simulink model "MIL4L3_SW6_V1_20220211"  (R2018b)
settings: Solver=FixedStepAuto  StartTime=0.0  StopTime=inf  FixedStep=0.001  RelTol=1e-3
PreLoadFcn:
  | A0_MILtest;
undefined symbols (not defined in the file or in its folder): Clb_ICADirect_LaneDisp_StateFive, Clb_ICADirect_LaneDisp_StateFour, Clb_ICADirect_LaneDisp_StateOne, Clb_ICADirect_LaneDisp_StateThree, Clb_ICADirect_LaneDisp_StateTwo, Clb_ICADirect_LaneDisp_StateZero, Clb_ICADirect_LaneDispSW, Clb_ICADirect_TrnLghtsCom_Switch, Clb_ICADirect_TrnLghtsCom_Value, Clb_ICADirect_TrnLghtsCrtl_Inhb, IMAP_Clb_ACU_Driver_Belt, IMAP_Clb_ACU_Driver_Belt_Over, IMAP_Clb_ACU_Passenger_Belt, IMAP_Clb_ACU_Passenger_Belt_Over, IMAP_Clb_ACU_RearLeft_Belt, IMAP_Clb_ACU_RearLeft_Belt_Over, IMAP_Clb_ACU_RearMiddle_Belt, IMAP_Clb_ACU_RearMiddle_Belt_Over, IMAP_Clb_ACU_RearRight_Belt, IMAP_Clb_ACU_RearRight_Belt_Over, IMAP_Clb_AEB_Switch, IMAP_Clb_AEB_Switch_Over, IMAP_Clb_ALC_TLC_Mode, IMAP_Clb_ALC_TLC_Mode_Over, IMAP_Clb_BCM_Battery_Voltage, IMAP_Clb_BCM_Battery_Voltage_Over, IMAP_Clb_BCM_BrakeLamp_State, IMAP_Clb_BCM_BrakeLamp_State_Over, IMAP_Clb_BCM_CHMSL_Status, IMAP_Clb_BCM_CHMSL_Status_Over, IMAP_Clb_BCM_Door_Lock_State, IMAP_Clb_BCM_Door_Lock_State_Over, IMAP_Clb_BCM_FrontWiper_State, IMAP_Clb_BCM_FrontWiper_State_Over, IMAP_Clb_BCM_FrontWiper_Switch, IMAP_Clb_BCM_FrontWiper_Switch_Over, IMAP_Clb_BCM_HazardLamp, IMAP_Clb_BCM_HazardLamp_Over, IMAP_Clb_BCM_HazardLamp_Switch, IMAP_Clb_BCM_HazardLamp_Switch_Over, IMAP_Clb_BCM_HighBeam_State, IMAP_Clb_BCM_HighBeam_State_Over, IMAP_Clb_BCM_Ignition_State, IMAP_Clb_BCM_Ignition_State_Over, IMAP_Clb_BCM_IHBC_Enabled, IMAP_Clb_BCM_IHBC_Enabled_Over, IMAP_Clb_BCM_Left_Light, IMAP_Clb_BCM_Left_Light_Over, IMAP_Clb_BCM_LeftTurn_Switch, IMAP_Clb_BCM_LeftTurn_Switch_Over, IMAP_Clb_BCM_LF_Door_State, IMAP_Clb_BCM_LF_Door_State_Over, IMAP_Clb_BCM_LowBeam_State, IMAP_Clb_BCM_LowBeam_State_Over, IMAP_Clb_BCM_LR_Door_State, IMAP_Clb_BCM_LR_Door_State_Over, IMAP_Clb_BCM_RF_Door_State, IMAP_Clb_BCM_RF_Door_State_Over, IMAP_Clb_BCM_Right_Light, IMAP_Clb_BCM_Right_Light_Over ... (+547)
libraries: CarMaker4SL x2153, simulink x292, dspstat3 x3, canmsglib x2, simulink_extras x1
(part 18 of 52)

== system MIL4L3_SW6_V1_20220211/CarMaker/VehicleControl/SDFADataLog/Subsystem97 ==
  BusCreator : BusCreator  Inputs=10
  Data Type Conversion{1..3,92} (4 alike) : DataTypeConversion  OutDataTypeStr=single
  Ground{,1..5} (6 alike) : Ground
  Read CM Dict1 : CarMaker4SL/Read CM Dict  xname=User.IO.Out.ReferencePoint_S0_002  xsync=off
  Read CM Dict2 : CarMaker4SL/Read CM Dict  xname=User.IO.Out.ReferencePoint_S0_003  xsync=off
  Read CM Dict3 : CarMaker4SL/Read CM Dict  xname=User.IO.Out.ReferencePoint_S0_004  xsync=off
  Read CM Dict5 : CarMaker4SL/Read CM Dict  xname=User.IO.Out.ReferencePoint_S0_001  xsync=off
  LBtar_ReferencePoint : Outport
  wires:
  Data Type Conversion3/1 -> BusCreator/4
  Data Type Conversion2/1 -> BusCreator/3
  Data Type Conversion92/1 -> BusCreator/1
  Data Type Conversion1/1 -> BusCreator/2
  Ground5/1 -> BusCreator/10
  Ground4/1 -> BusCreator/9
  Ground3/1 -> BusCreator/8
  Ground2/1 -> BusCreator/7
  Ground1/1 -> BusCreator/6
  Ground/1 -> BusCreator/5
  Read CM Dict5/1 -> Data Type Conversion92/1
  Read CM Dict1/1 -> Data Type Conversion1/1
  Read CM Dict2/1 -> Data Type Conversion2/1
  Read CM Dict3/1 -> Data Type Conversion3/1
  BusCreator/1 -> LBtar_ReferencePoint/1

== system MIL4L3_SW6_V1_20220211/CarMaker/VehicleControl/SDFADataLog/Subsystem98 ==
  BusCreator : BusCreator  Inputs=10
  Data Type Conversion{1..3,92} (4 alike) : DataTypeConversion  OutDataTypeStr=single
  Ground{,1..5} (6 alike) : Ground
  Read CM Dict1 : CarMaker4SL/Read CM Dict  xname=User.IO.Out.MovingState_S0_002  xsync=off
  Read CM Dict2 : CarMaker4SL/Read CM Dict  xname=User.IO.Out.MovingState_S0_003  xsync=off
  Read CM Dict3 : CarMaker4SL/Read CM Dict  xname=User.IO.Out.MovingState_S0_004  xsync=off
  Read CM Dict5 : CarMaker4SL/Read CM Dict  xname=User.IO.Out.MovingState_S0_001  xsync=off
  LBtar_MovingState : Outport
  wires:
  Data Type Conversion92/1 -> BusCreator/1
  Data Type Conversion2/1 -> BusCreator/3
  Data Type Conversion3/1 -> BusCreator/4
  Data Type Conversion1/1 -> BusCreator/2
  BusCreator/1 -> LBtar_MovingState/1
  Read CM Dict3/1 -> Data Type Conversion3/1
  Read CM Dict2/1 -> Data Type Conversion2/1
  Read CM Dict1/1 -> Data Type Conversion1/1
  Read CM Dict5/1 -> Data Type Conversion92/1
  Ground/1 -> BusCreator/5
  Ground1/1 -> BusCreator/6
  Ground2/1 -> BusCreator/7
  Ground3/1 -> BusCreator/8
  Ground4/1 -> BusCreator/9
  Ground5/1 -> BusCreator/10

== system MIL4L3_SW6_V1_20220211/CarMaker/VehicleControl/SwitchForRealECU_ACC_Brake/PI Control ==
  Add : Sum
  Constant : Constant  Value=0
  Constant1 : Constant  Value=0
  Constant2 : Constant  Value=0
  Define CM Dict5 : CarMaker4SL/Define CM Dict  xname=User.IO.In.P_gain  xmono=off  xtype=Double4  xdvaplace=IO_In  xnstates=0  xfirststate=0  xinitial=-0.06
  Define CM Dict6 : CarMaker4SL/Define CM Dict  xname=User.IO.In.I_gain  xmono=off  xtype=Double4  xdvaplace=IO_In  xnstates=0  xfirststate=0  xinitial=-0.03
  Delta ax : Sum  Inputs=+-
  Memory : Memory
  Product : Product
  Product1 : Product
  Read CM Dict1 : CarMaker4SL/Read CM Dict  xname=User.IO.In.P_gain  xsync=off
  Read CM Dict2 : CarMaker4SL/Read CM Dict  xname=User.IO.In.I_gain  xsync=off
  Read CM Dict7 : CarMaker4SL/Read CM Dict  xname=Car.ax  xsync=off
  Saturation : Saturate  UpperLimit=1  LowerLimit=0
  Saturation1 : Saturate  UpperLimit=1  LowerLimit=0
  Sum : Sum  Inputs=|++
  Switch : Switch  Criteria=u2 > Threshold
  Switch1 : Switch  Criteria=u2 > Threshold
  Switch2 : Switch  Criteria=u2 > Threshold
  Out1 : Outport
  wires:
  [ADAS_DecelerationSet] -> Switch/1
  Switch/1 -> Delta ax/1
  Delta ax/1 -> Product1/1, Product/2
  Add/1 -> Saturation1/1
  Product/1 -> Add/1
  Product1/1 -> Sum/1
  Sum/1 -> Memory/1, Switch2/1
  Memory/1 -> Saturation/1
  Saturation/1 -> Sum/2
  Read CM Dict1/1 -> Product/1
  Read CM Dict2/1 -> Product1/2
  [MDD_Decelerationcontrol_request] -> Switch1/2, Switch2/2, Switch/2
  Read CM Dict7/1 -> Switch1/1
  Constant/1 -> Switch1/3
  Switch1/1 -> Delta ax/2
  Switch2/1 -> Add/2
  Constant1/1 -> Switch2/3
  Saturation1/1 -> Out1/1
  Constant2/1 -> Switch/3

== system MIL4L3_SW6_V1_20220211/CarMaker/VehicleControl/SwitchForRealECU_ACC_Gas/PI Control ==
  In1 : Inport
  Add : Sum
  Compare To Constant1 : simulink/Logic and Bit Operations/Compare To Constant  relop===  const=1  OutDataTypeStr=boolean
  Constant : Constant  Value=0
  Constant1 : Constant  Value=0
  Define CM Dict5 : CarMaker4SL/Define CM Dict  xname=User.IO.In.EngTrqManualC  xmono=off  xtype=Double4  xdvaplace=IO_In  xnstates=0  xfirststate=0  xinitial=1
  Delta Tq : Sum  Inputs=+-
  Gain : Gain  Gain=-1/500
  Gain1 : Gain  Gain=-1/500
  Gain2 : Gain  Gain=0.95
  Gain3 : Gain  Gain=0.98
  Gain4 : Gain
  Memory : Memory
  Product : Product
  Product1 : Product
  Product2 : Product  Inputs=3
  Read CM Dict1 : CarMaker4SL/Read CM Dict  xname=User.IO.In.P_gain  xsync=off
  Read CM Dict11 : CarMaker4SL/Read CM Dict  xname=PT.Engine.Trq  xsync=off
  Read CM Dict2 : CarMaker4SL/Read CM Dict  xname=User.IO.In.I_gain  xsync=off
  Read CM Dict3 : CarMaker4SL/Read CM Dict  xname=User.IO.In.ADAS_PowerWheelTorqueActiveReq  xsync=off
  Read CM Dict5 : CarMaker4SL/Read CM Dict  xname=User.IO.In.EngTrqManualC  xsync=off
  Saturation : Saturate  UpperLimit=1  LowerLimit=0
  Saturation1 : Saturate  UpperLimit=1  LowerLimit=0
  Subsystem1 : Subsystem
  Sum : Sum  Inputs=|++
  Switch1 : Switch  Criteria=u2 > Threshold  Threshold=0.5
  Switch2 : Switch  Criteria=u2 > Threshold  Threshold=0.5
  Out1 : Outport
  wires:
  In1/1 -> Delta Tq/1
  Delta Tq/1 -> Product1/1, Product/2
  Product/1 -> Add/1
  Product1/1 -> Sum/1
  Sum/1 -> Memory/1, Switch2/1
  Memory/1 -> Saturation/1
  Saturation/1 -> Sum/2
  Read CM Dict1/1 -> Gain/1
  Compare To Constant1/1 -> Switch2/2, Switch1/2
  Constant/1 -> Switch1/3
  Switch1/1 -> Delta Tq/2
  Switch2/1 -> Add/2
  Constant1/1 -> Switch2/3
  Saturation1/1 -> Out1/1
  Gain/1 -> Product/1
  Read CM Dict3/1 -> Compare To Constant1/1
  Product2/1 -> Switch1/1
  Read CM Dict2/1 -> Gain1/1
  Gain1/1 -> Product1/2
  Add/1 -> Saturation1/1
  Read CM Dict11/1 -> Product2/2
  Gain3/1 -> Product2/3
  Read CM Dict5/1 -> Product2/1
  Subsystem1/1(TCU_AGB_position) -> Gain2/1  "Ratio"
  Gain2/1 -> Gain4/1
  Gain4/1 -> Gain3/1

== system MIL4L3_SW6_V1_20220211/CarMaker/VehicleControl/SwitchForRealECU_Steering_Angle/Subsystem1 ==
  In1 : Inport
  Constant : Constant  Value=0
  Dead Zone : DeadZone  LowerValue=0  UpperValue=0  SaturateOnIntegerOverflow=on
  Rate Limiter : RateLimiter  SampleTimeMode=inherited
  Subtract : Sum  Inputs=+-
  Transfer Fcn : TransferFcn  Denominator=[0.002 1]
  Out1 : Outport
  wires:
  Constant/1 -> Subtract/2
  Rate Limiter/1 -> Subtract/1
  Transfer Fcn/1 -> Dead Zone/1
  Subtract/1 -> Transfer Fcn/1
  In1/1 -> Rate Limiter/1
  Dead Zone/1 -> Out1/1

== system MIL4L3_SW6_V1_20220211/CarMaker/VehicleControl/Traffic Attribution Define1/T00 ==
  Define CM Dict 10 : CarMaker4SL/Define CM Dict  xname=User.IO.Out.T00.class  xmono=off  xtype=Double4  xdvaplace=IO_Out  xnstates=0  xfirststate=0  xinitial=1
  Define CM Dict 11 : CarMaker4SL/Define CM Dict  xname=User.IO.Out.T00.ObjectInfo  xmono=off  xtype=Double4  xdvaplace=IO_Out  xnstates=0  xfirststate=0  xinitial=2
  Define CM Dict 12 : CarMaker4SL/Define CM Dict  xname=User.IO.Out.T00.ClassHighestProb  xmono=off  xtype=Double4  xdvaplace=IO_Out  xnstates=0  xfirststate=0  xinitial=2
  Define CM Dict 13 : CarMaker4SL/Define CM Dict  xname=User.IO.Out.T00.status  xmono=off  xtype=Double4  xdvaplace=IO_Out  xnstates=0  xfirststate=0  xinitial=0
  Define CM Dict 14 : CarMaker4SL/Define CM Dict  xname=User.IO.Out.T00.probility  xmono=off  xtype=Double4  xdvaplace=IO_Out  xnstates=0  xfirststate=0  xinitial=0.9
  Define CM Dict 15 : CarMaker4SL/Define CM Dict  xname=User.IO.Out.T00.power  xmono=off  xtype=Double4  xdvaplace=IO_Out  xnstates=0  xfirststate=0  xinitial=90
  Define CM Dict 16 : CarMaker4SL/Define CM Dict  xname=User.IO.Out.T00.Turn_signal  xmono=off  xtype=Double4  xdvaplace=IO_Out  xnstates=0  xfirststate=0  xinitial=0
  Define CM Dict 17 : CarMaker4SL/Define CM Dict  xname=User.IO.Out.T00.BrakeLight  xmono=off  xtype=Double4  xdvaplace=IO_Out  xnstates=0  xfirststate=0  xinitial=0
  Define CM Dict 9 : CarMaker4SL/Define CM Dict  xname=User.IO.Out.T00.ExistenceProbability  xmono=off  xtype=Double4  xdvaplace=IO_Out  xnstates=0  xfirststate=0  xinitial=0.95
  Define CM Dict5 : CarMaker4SL/Define CM Dict  xname=User.IO.Out.T00.longdistance  xmono=off  xtype=Double4  xdvaplace=None  xnstates=0  xfirststate=0  xinitial=0
  Define CM Dict6 : CarMaker4SL/Define CM Dict  xname=User.IO.Out.T00.RelVxValid  xmono=off  xtype=Double4  xdvaplace=None  xnstates=0  xfirststate=0  xinitial=1
  Define CM Dict7 : CarMaker4SL/Define CM Dict  xname=User.IO.Out.T00.RelVyValid  xmono=off  xtype=Double4  xdvaplace=None  xnstates=0  xfirststate=0  xinitial=1
  Define CM Dict8 : CarMaker4SL/Define CM Dict  xname=User.IO.Out.T00.TypeProb  xmono=off  xtype=Double4  xdvaplace=None  xnstates=0  xfirststate=0  xinitial=1
  Define CM Dict9 : CarMaker4SL/Define CM Dict  xname=User.IO.Out.T00.Measured  xmono=off  xtype=Double4  xdvaplace=None  xnstates=0  xfirststate=0  xinitial=2

== system MIL4L3_SW6_V1_20220211/CarMaker/VehicleControl/Traffic Attribution Define1/T01 ==
  Define CM Dict 0 : CarMaker4SL/Define CM Dict  xname=User.IO.Out.T01.ExistenceProbability  xmono=off  xtype=Double4  xdvaplace=IO_Out  xnstates=0  xfirststate=0  xinitial=0.95
  Define CM Dict 1 : CarMaker4SL/Define CM Dict  xname=User.IO.Out.T01.class  xmono=off  xtype=Double4  xdvaplace=IO_Out  xnstates=0  xfirststate=0  xinitial=1
  Define CM Dict 2 : CarMaker4SL/Define CM Dict  xname=User.IO.Out.T01.ObjectInfo  xmono=off  xtype=Double4  xdvaplace=IO_Out  xnstates=0  xfirststate=0  xinitial=2
  Define CM Dict 3 : CarMaker4SL/Define CM Dict  xname=User.IO.Out.T01.ClassHighestProb  xmono=off  xtype=Double4  xdvaplace=IO_Out  xnstates=0  xfirststate=0  xinitial=2
  Define CM Dict 4 : CarMaker4SL/Define CM Dict  xname=User.IO.Out.T01.status  xmono=off  xtype=Double4  xdvaplace=IO_Out  xnstates=0  xfirststate=0  xinitial=0
  Define CM Dict 5 : CarMaker4SL/Define CM Dict  xname=User.IO.Out.T01.probility  xmono=off  xtype=Double4  xdvaplace=IO_Out  xnstates=0  xfirststate=0  xinitial=0.9
  Define CM Dict 6 : CarMaker4SL/Define CM Dict  xname=User.IO.Out.T01.power  xmono=off  xtype=Double4  xdvaplace=IO_Out  xnstates=0  xfirststate=0  xinitial=90
  Define CM Dict 7 : CarMaker4SL/Define CM Dict  xname=User.IO.Out.T01.Turn_signal  xmono=off  xtype=Double4  xdvaplace=IO_Out  xnstates=0  xfirststate=0  xinitial=0
  Define CM Dict 8 : CarMaker4SL/Define CM Dict  xname=User.IO.Out.T01.BrakeLight  xmono=off  xtype=Double4  xdvaplace=IO_Out  xnstates=0  xfirststate=0  xinitial=0
  Define CM Dict5 : CarMaker4SL/Define CM Dict  xname=User.IO.Out.T01.longdistance  xmono=off  xtype=Double4  xdvaplace=None  xnstates=0  xfirststate=0  xinitial=0
  Define CM Dict6 : CarMaker4SL/Define CM Dict  xname=User.IO.Out.T01.RelVxValid  xmono=off  xtype=Double4  xdvaplace=None  xnstates=0  xfirststate=0  xinitial=1
  Define CM Dict7 : CarMaker4SL/Define CM Dict  xname=User.IO.Out.T01.RelVyValid  xmono=off  xtype=Double4  xdvaplace=None  xnstates=0  xfirststate=0  xinitial=1
  Define CM Dict8 : CarMaker4SL/Define CM Dict  xname=User.IO.Out.T01.TypeProb  xmono=off  xtype=Double4  xdvaplace=None  xnstates=0  xfirststate=0  xinitial=1
  Define CM Dict9 : CarMaker4SL/Define CM Dict  xname=User.IO.Out.T01.Measured  xmono=off  xtype=Double4  xdvaplace=None  xnstates=0  xfirststate=0  xinitial=2

== system MIL4L3_SW6_V1_20220211/CarMaker/VehicleControl/Traffic Attribution Define1/T02 ==
  Define CM Dict 0 : CarMaker4SL/Define CM Dict  xname=User.IO.Out.T02.ExistenceProbability  xmono=off  xtype=Double4  xdvaplace=IO_Out  xnstates=0  xfirststate=0  xinitial=0.95
  Define CM Dict 1 : CarMaker4SL/Define CM Dict  xname=User.IO.Out.T02.class  xmono=off  xtype=Double4  xdvaplace=IO_Out  xnstates=0  xfirststate=0  xinitial=1
  Define CM Dict 2 : CarMaker4SL/Define CM Dict  xname=User.IO.Out.T02.ObjectInfo  xmono=off  xtype=Double4  xdvaplace=IO_Out  xnstates=0  xfirststate=0  xinitial=2
  Define CM Dict 3 : CarMaker4SL/Define CM Dict  xname=User.IO.Out.T02.ClassHighestProb  xmono=off  xtype=Double4  xdvaplace=IO_Out  xnstates=0  xfirststate=0  xinitial=2
  Define CM Dict 4 : CarMaker4SL/Define CM Dict  xname=User.IO.Out.T02.status  xmono=off  xtype=Double4  xdvaplace=IO_Out  xnstates=0  xfirststate=0  xinitial=0
  Define CM Dict 5 : CarMaker4SL/Define CM Dict  xname=User.IO.Out.T02.probility  xmono=off  xtype=Double4  xdvaplace=IO_Out  xnstates=0  xfirststate=0  xinitial=0.9
  Define CM Dict 6 : CarMaker4SL/Define CM Dict  xname=User.IO.Out.T02.power  xmono=off  xtype=Double4  xdvaplace=IO_Out  xnstates=0  xfirststate=0  xinitial=90
  Define CM Dict 7 : CarMaker4SL/Define CM Dict  xname=User.IO.Out.T02.Turn_signal  xmono=off  xtype=Double4  xdvaplace=IO_Out  xnstates=0  xfirststate=0  xinitial=0
  Define CM Dict 8 : CarMaker4SL/Define CM Dict  xname=User.IO.Out.T02.BrakeLight  xmono=off  xtype=Double4  xdvaplace=IO_Out  xnstates=0  xfirststate=0  xinitial=0
  Define CM Dict5 : CarMaker4SL/Define CM Dict  xname=User.IO.Out.T02.longdistance  xmono=off  xtype=Double4  xdvaplace=None  xnstates=0  xfirststate=0  xinitial=0
  Define CM Dict6 : CarMaker4SL/Define CM Dict  xname=User.IO.Out.T02.RelVxValid  xmono=off  xtype=Double4  xdvaplace=None  xnstates=0  xfirststate=0  xinitial=1
  Define CM Dict7 : CarMaker4SL/Define CM Dict  xname=User.IO.Out.T02.RelVyValid  xmono=off  xtype=Double4  xdvaplace=None  xnstates=0  xfirststate=0  xinitial=1
  Define CM Dict8 : CarMaker4SL/Define CM Dict  xname=User.IO.Out.T02.TypeProb  xmono=off  xtype=Double4  xdvaplace=None  xnstates=0  xfirststate=0  xinitial=1
  Define CM Dict9 : CarMaker4SL/Define CM Dict  xname=User.IO.Out.T02.Measured  xmono=off  xtype=Double4  xdvaplace=None  xnstates=0  xfirststate=0  xinitial=2

== system MIL4L3_SW6_V1_20220211/CarMaker/VehicleControl/Traffic Attribution Define1/T03 ==
  Define CM Dict 0 : CarMaker4SL/Define CM Dict  xname=User.IO.Out.T03.ExistenceProbability  xmono=off  xtype=Double4  xdvaplace=IO_Out  xnstates=0  xfirststate=0  xinitial=0.95
  Define CM Dict 1 : CarMaker4SL/Define CM Dict  xname=User.IO.Out.T03.class  xmono=off  xtype=Double4  xdvaplace=IO_Out  xnstates=0  xfirststate=0  xinitial=1
  Define CM Dict 2 : CarMaker4SL/Define CM Dict  xname=User.IO.Out.T03.ObjectInfo  xmono=off  xtype=Double4  xdvaplace=IO_Out  xnstates=0  xfirststate=0  xinitial=2
  Define CM Dict 3 : CarMaker4SL/Define CM Dict  xname=User.IO.Out.T03.ClassHighestProb  xmono=off  xtype=Double4  xdvaplace=IO_Out  xnstates=0  xfirststate=0  xinitial=2
  Define CM Dict 4 : CarMaker4SL/Define CM Dict  xname=User.IO.Out.T03.status  xmono=off  xtype=Double4  xdvaplace=IO_Out  xnstates=0  xfirststate=0  xinitial=0
  Define CM Dict 5 : CarMaker4SL/Define CM Dict  xname=User.IO.Out.T03.probility  xmono=off  xtype=Double4  xdvaplace=IO_Out  xnstates=0  xfirststate=0  xinitial=0.9
  Define CM Dict 6 : CarMaker4SL/Define CM Dict  xname=User.IO.Out.T03.power  xmono=off  xtype=Double4  xdvaplace=IO_Out  xnstates=0  xfirststate=0  xinitial=90
  Define CM Dict 7 : CarMaker4SL/Define CM Dict  xname=User.IO.Out.T03.Turn_signal  xmono=off  xtype=Double4  xdvaplace=IO_Out  xnstates=0  xfirststate=0  xinitial=0
  Define CM Dict 8 : CarMaker4SL/Define CM Dict  xname=User.IO.Out.T03.BrakeLight  xmono=off  xtype=Double4  xdvaplace=IO_Out  xnstates=0  xfirststate=0  xinitial=0
  Define CM Dict5 : CarMaker4SL/Define CM Dict  xname=User.IO.Out.T03.longdistance  xmono=off  xtype=Double4  xdvaplace=None  xnstates=0  xfirststate=0  xinitial=0
  Define CM Dict6 : CarMaker4SL/Define CM Dict  xname=User.IO.Out.T03.RelVxValid  xmono=off  xtype=Double4  xdvaplace=None  xnstates=0  xfirststate=0  xinitial=1
  Define CM Dict7 : CarMaker4SL/Define CM Dict  xname=User.IO.Out.T03.RelVyValid  xmono=off  xtype=Double4  xdvaplace=None  xnstates=0  xfirststate=0  xinitial=1
  Define CM Dict8 : CarMaker4SL/Define CM Dict  xname=User.IO.Out.T03.TypeProb  xmono=off  xtype=Double4  xdvaplace=None  xnstates=0  xfirststate=0  xinitial=1
  Define CM Dict9 : CarMaker4SL/Define CM Dict  xname=User.IO.Out.T03.Measured  xmono=off  xtype=Double4  xdvaplace=None  xnstates=0  xfirststate=0  xinitial=2

== system MIL4L3_SW6_V1_20220211/CarMaker/VehicleControl/Traffic Attribution Define1/T04 ==
  Define CM Dict 0 : CarMaker4SL/Define CM Dict  xname=User.IO.Out.T04.ExistenceProbability  xmono=off  xtype=Double4  xdvaplace=IO_Out  xnstates=0  xfirststate=0  xinitial=0.95
  Define CM Dict 1 : CarMaker4SL/Define CM Dict  xname=User.IO.Out.T04.class  xmono=off  xtype=Double4  xdvaplace=IO_Out  xnstates=0  xfirststate=0  xinitial=1
  Define CM Dict 2 : CarMaker4SL/Define CM Dict  xname=User.IO.Out.T04.ObjectInfo  xmono=off  xtype=Double4  xdvaplace=IO_Out  xnstates=0  xfirststate=0  xinitial=2
  Define CM Dict 3 : CarMaker4SL/Define CM Dict  xname=User.IO.Out.T04.ClassHighestProb  xmono=off  xtype=Double4  xdvaplace=IO_Out  xnstates=0  xfirststate=0  xinitial=2
  Define CM Dict 4 : CarMaker4SL/Define CM Dict  xname=User.IO.Out.T04.status  xmono=off  xtype=Double4  xdvaplace=IO_Out  xnstates=0  xfirststate=0  xinitial=0
  Define CM Dict 5 : CarMaker4SL/Define CM Dict  xname=User.IO.Out.T04.probility  xmono=off  xtype=Double4  xdvaplace=IO_Out  xnstates=0  xfirststate=0  xinitial=0.9
  Define CM Dict 6 : CarMaker4SL/Define CM Dict  xname=User.IO.Out.T04.power  xmono=off  xtype=Double4  xdvaplace=IO_Out  xnstates=0  xfirststate=0  xinitial=90
  Define CM Dict 7 : CarMaker4SL/Define CM Dict  xname=User.IO.Out.T04.Turn_signal  xmono=off  xtype=Double4  xdvaplace=IO_Out  xnstates=0  xfirststate=0  xinitial=0
  Define CM Dict 8 : CarMaker4SL/Define CM Dict  xname=User.IO.Out.T04.BrakeLight  xmono=off  xtype=Double4  xdvaplace=IO_Out  xnstates=0  xfirststate=0  xinitial=0
  Define CM Dict5 : CarMaker4SL/Define CM Dict  xname=User.IO.Out.T04.longdistance  xmono=off  xtype=Double4  xdvaplace=None  xnstates=0  xfirststate=0  xinitial=0
  Define CM Dict6 : CarMaker4SL/Define CM Dict  xname=User.IO.Out.T04.RelVxValid  xmono=off  xtype=Double4  xdvaplace=None  xnstates=0  xfirststate=0  xinitial=1
  Define CM Dict7 : CarMaker4SL/Define CM Dict  xname=User.IO.Out.T04.RelVyValid  xmono=off  xtype=Double4  xdvaplace=None  xnstates=0  xfirststate=0  xinitial=1
  Define CM Dict8 : CarMaker4SL/Define CM Dict  xname=User.IO.Out.T04.TypeProb  xmono=off  xtype=Double4  xdvaplace=None  xnstates=0  xfirststate=0  xinitial=1
  Define CM Dict9 : CarMaker4SL/Define CM Dict  xname=User.IO.Out.T04.Measured  xmono=off  xtype=Double4  xdvaplace=None  xnstates=0  xfirststate=0  xinitial=2

== system MIL4L3_SW6_V1_20220211/CarMaker/VehicleControl/Traffic Attribution Define1/T05 ==
  Define CM Dict 0 : CarMaker4SL/Define CM Dict  xname=User.IO.Out.T05.ExistenceProbability  xmono=off  xtype=Double4  xdvaplace=IO_Out  xnstates=0  xfirststate=0  xinitial=0.95
  Define CM Dict 1 : CarMaker4SL/Define CM Dict  xname=User.IO.Out.T05.class  xmono=off  xtype=Double4  xdvaplace=IO_Out  xnstates=0  xfirststate=0  xinitial=1
  Define CM Dict 2 : CarMaker4SL/Define CM Dict  xname=User.IO.Out.T05.ObjectInfo  xmono=off  xtype=Double4  xdvaplace=IO_Out  xnstates=0  xfirststate=0  xinitial=2
  Define CM Dict 3 : CarMaker4SL/Define CM Dict  xname=User.IO.Out.T05.ClassHighestProb  xmono=off  xtype=Double4  xdvaplace=IO_Out  xnstates=0  xfirststate=0  xinitial=2
  Define CM Dict 4 : CarMaker4SL/Define CM Dict  xname=User.IO.Out.T05.status  xmono=off  xtype=Double4  xdvaplace=IO_Out  xnstates=0  xfirststate=0  xinitial=0
  Define CM Dict 5 : CarMaker4SL/Define CM Dict  xname=User.IO.Out.T05.probility  xmono=off  xtype=Double4  xdvaplace=IO_Out  xnstates=0  xfirststate=0  xinitial=0.9
  Define CM Dict 6 : CarMaker4SL/Define CM Dict  xname=User.IO.Out.T05.power  xmono=off  xtype=Double4  xdvaplace=IO_Out  xnstates=0  xfirststate=0  xinitial=90
  Define CM Dict 7 : CarMaker4SL/Define CM Dict  xname=User.IO.Out.T05.Turn_signal  xmono=off  xtype=Double4  xdvaplace=IO_Out  xnstates=0  xfirststate=0  xinitial=0
  Define CM Dict 8 : CarMaker4SL/Define CM Dict  xname=User.IO.Out.T05.BrakeLight  xmono=off  xtype=Double4  xdvaplace=IO_Out  xnstates=0  xfirststate=0  xinitial=0
  Define CM Dict5 : CarMaker4SL/Define CM Dict  xname=User.IO.Out.T05.longdistance  xmono=off  xtype=Double4  xdvaplace=None  xnstates=0  xfirststate=0  xinitial=0
  Define CM Dict6 : CarMaker4SL/Define CM Dict  xname=User.IO.Out.T05.RelVxValid  xmono=off  xtype=Double4  xdvaplace=None  xnstates=0  xfirststate=0  xinitial=1
  Define CM Dict7 : CarMaker4SL/Define CM Dict  xname=User.IO.Out.T05.RelVyValid  xmono=off  xtype=Double4  xdvaplace=None  xnstates=0  xfirststate=0  xinitial=1
  Define CM Dict8 : CarMaker4SL/Define CM Dict  xname=User.IO.Out.T05.TypeProb  xmono=off  xtype=Double4  xdvaplace=None  xnstates=0  xfirststate=0  xinitial=1
  Define CM Dict9 : CarMaker4SL/Define CM Dict  xname=User.IO.Out.T05.Measured  xmono=off  xtype=Double4  xdvaplace=None  xnstates=0  xfirststate=0  xinitial=2

== system MIL4L3_SW6_V1_20220211/CarMaker/VehicleControl/Traffic Attribution Define1/T06 ==
  Define CM Dict 0 : CarMaker4SL/Define CM Dict  xname=User.IO.Out.T06.ExistenceProbability  xmono=off  xtype=Double4  xdvaplace=IO_Out  xnstates=0  xfirststate=0  xinitial=0.95
  Define CM Dict 1 : CarMaker4SL/Define CM Dict  xname=User.IO.Out.T06.class  xmono=off  xtype=Double4  xdvaplace=IO_Out  xnstates=0  xfirststate=0  xinitial=1
  Define CM Dict 2 : CarMaker4SL/Define CM Dict  xname=User.IO.Out.T06.ObjectInfo  xmono=off  xtype=Double4  xdvaplace=IO_Out  xnstates=0  xfirststate=0  xinitial=2
  Define CM Dict 3 : CarMaker4SL/Define CM Dict  xname=User.IO.Out.T06.ClassHighestProb  xmono=off  xtype=Double4  xdvaplace=IO_Out  xnstates=0  xfirststate=0  xinitial=2
  Define CM Dict 4 : CarMaker4SL/Define CM Dict  xname=User.IO.Out.T06.status  xmono=off  xtype=Double4  xdvaplace=IO_Out  xnstates=0  xfirststate=0  xinitial=0
  Define CM Dict 5 : CarMaker4SL/Define CM Dict  xname=User.IO.Out.T06.probility  xmono=off  xtype=Double4  xdvaplace=IO_Out  xnstates=0  xfirststate=0  xinitial=0.9
  Define CM Dict 6 : CarMaker4SL/Define CM Dict  xname=User.IO.Out.T06.power  xmono=off  xtype=Double4  xdvaplace=IO_Out  xnstates=0  xfirststate=0  xinitial=90
  Define CM Dict 7 : CarMaker4SL/Define CM Dict  xname=User.IO.Out.T06.Turn_signal  xmono=off  xtype=Double4  xdvaplace=IO_Out  xnstates=0  xfirststate=0  xinitial=0
  Define CM Dict 8 : CarMaker4SL/Define CM Dict  xname=User.IO.Out.T06.BrakeLight  xmono=off  xtype=Double4  xdvaplace=IO_Out  xnstates=0  xfirststate=0  xinitial=0
  Define CM Dict5 : CarMaker4SL/Define CM Dict  xname=User.IO.Out.T06.longdistance  xmono=off  xtype=Double4  xdvaplace=None  xnstates=0  xfirststate=0  xinitial=0
  Define CM Dict6 : CarMaker4SL/Define CM Dict  xname=User.IO.Out.T06.RelVxValid  xmono=off  xtype=Double4  xdvaplace=None  xnstates=0  xfirststate=0  xinitial=1
  Define CM Dict7 : CarMaker4SL/Define CM Dict  xname=User.IO.Out.T06.RelVyValid  xmono=off  xtype=Double4  xdvaplace=None  xnstates=0  xfirststate=0  xinitial=1
  Define CM Dict8 : CarMaker4SL/Define CM Dict  xname=User.IO.Out.T06.TypeProb  xmono=off  xtype=Double4  xdvaplace=None  xnstates=0  xfirststate=0  xinitial=1
  Define CM Dict9 : CarMaker4SL/Define CM Dict  xname=User.IO.Out.T06.Measured  xmono=off  xtype=Double4  xdvaplace=None  xnstates=0  xfirststate=0  xinitial=2

== system MIL4L3_SW6_V1_20220211/CarMaker/VehicleControl/Traffic Attribution Define1/T07 ==
  Define CM Dict 0 : CarMaker4SL/Define CM Dict  xname=User.IO.Out.T07.ExistenceProbability  xmono=off  xtype=Double4  xdvaplace=IO_Out  xnstates=0  xfirststate=0  xinitial=0.95
  Define CM Dict 1 : CarMaker4SL/Define CM Dict  xname=User.IO.Out.T07.class  xmono=off  xtype=Double4  xdvaplace=IO_Out  xnstates=0  xfirststate=0  xinitial=1
  Define CM Dict 2 : CarMaker4SL/Define CM Dict  xname=User.IO.Out.T07.ObjectInfo  xmono=off  xtype=Double4  xdvaplace=IO_Out  xnstates=0  xfirststate=0  xinitial=2
  Define CM Dict 3 : CarMaker4SL/Define CM Dict  xname=User.IO.Out.T07.ClassHighestProb  xmono=off  xtype=Double4  xdvaplace=IO_Out  xnstates=0  xfirststate=0  xinitial=2
  Define CM Dict 4 : CarMaker4SL/Define CM Dict  xname=User.IO.Out.T07.status  xmono=off  xtype=Double4  xdvaplace=IO_Out  xnstates=0  xfirststate=0  xinitial=0
  Define CM Dict 5 : CarMaker4SL/Define CM Dict  xname=User.IO.Out.T07.probility  xmono=off  xtype=Double4  xdvaplace=IO_Out  xnstates=0  xfirststate=0  xinitial=0.9
  Define CM Dict 6 : CarMaker4SL/Define CM Dict  xname=User.IO.Out.T07.power  xmono=off  xtype=Double4  xdvaplace=IO_Out  xnstates=0  xfirststate=0  xinitial=90
  Define CM Dict 7 : CarMaker4SL/Define CM Dict  xname=User.IO.Out.T07.Turn_signal  xmono=off  xtype=Double4  xdvaplace=IO_Out  xnstates=0  xfirststate=0  xinitial=0
  Define CM Dict 8 : CarMaker4SL/Define CM Dict  xname=User.IO.Out.T07.BrakeLight  xmono=off  xtype=Double4  xdvaplace=IO_Out  xnstates=0  xfirststate=0  xinitial=0
  Define CM Dict5 : CarMaker4SL/Define CM Dict  xname=User.IO.Out.T07.longdistance  xmono=off  xtype=Double4  xdvaplace=None  xnstates=0  xfirststate=0  xinitial=0
  Define CM Dict6 : CarMaker4SL/Define CM Dict  xname=User.IO.Out.T07.RelVxValid  xmono=off  xtype=Double4  xdvaplace=None  xnstates=0  xfirststate=0  xinitial=1
  Define CM Dict7 : CarMaker4SL/Define CM Dict  xname=User.IO.Out.T07.RelVyValid  xmono=off  xtype=Double4  xdvaplace=None  xnstates=0  xfirststate=0  xinitial=1
  Define CM Dict8 : CarMaker4SL/Define CM Dict  xname=User.IO.Out.T07.TypeProb  xmono=off  xtype=Double4  xdvaplace=None  xnstates=0  xfirststate=0  xinitial=1
  Define CM Dict9 : CarMaker4SL/Define CM Dict  xname=User.IO.Out.T07.Measured  xmono=off  xtype=Double4  xdvaplace=None  xnstates=0  xfirststate=0  xinitial=2

== system MIL4L3_SW6_V1_20220211/CarMaker/VehicleControl/Traffic Attribution Define1/T08 ==
  Define CM Dict 0 : CarMaker4SL/Define CM Dict  xname=User.IO.Out.T08.ExistenceProbability  xmono=off  xtype=Double4  xdvaplace=IO_Out  xnstates=0  xfirststate=0  xinitial=0.95
  Define CM Dict 1 : CarMaker4SL/Define CM Dict  xname=User.IO.Out.T08.class  xmono=off  xtype=Double4  xdvaplace=IO_Out  xnstates=0  xfirststate=0  xinitial=1
  Define CM Dict 2 : CarMaker4SL/Define CM Dict  xname=User.IO.Out.T08.ObjectInfo  xmono=off  xtype=Double4  xdvaplace=IO_Out  xnstates=0  xfirststate=0  xinitial=2
  Define CM Dict 3 : CarMaker4SL/Define CM Dict  xname=User.IO.Out.T08.ClassHighestProb  xmono=off  xtype=Double4  xdvaplace=IO_Out  xnstates=0  xfirststate=0  xinitial=2
  Define CM Dict 4 : CarMaker4SL/Define CM Dict  xname=User.IO.Out.T08.status  xmono=off  xtype=Double4  xdvaplace=IO_Out  xnstates=0  xfirststate=0  xinitial=0
  Define CM Dict 5 : CarMaker4SL/Define CM Dict  xname=User.IO.Out.T08.probility  xmono=off  xtype=Double4  xdvaplace=IO_Out  xnstates=0  xfirststate=0  xinitial=0.9
  Define CM Dict 6 : CarMaker4SL/Define CM Dict  xname=User.IO.Out.T08.power  xmono=off  xtype=Double4  xdvaplace=IO_Out  xnstates=0  xfirststate=0  xinitial=90
  Define CM Dict 7 : CarMaker4SL/Define CM Dict  xname=User.IO.Out.T08.Turn_signal  xmono=off  xtype=Double4  xdvaplace=IO_Out  xnstates=0  xfirststate=0  xinitial=0
  Define CM Dict 8 : CarMaker4SL/Define CM Dict  xname=User.IO.Out.T08.BrakeLight  xmono=off  xtype=Double4  xdvaplace=IO_Out  xnstates=0  xfirststate=0  xinitial=0
  Define CM Dict5 : CarMaker4SL/Define CM Dict  xname=User.IO.Out.T08.longdistance  xmono=off  xtype=Double4  xdvaplace=None  xnstates=0  xfirststate=0  xinitial=0
  Define CM Dict6 : CarMaker4SL/Define CM Dict  xname=User.IO.Out.T08.RelVxValid  xmono=off  xtype=Double4  xdvaplace=None  xnstates=0  xfirststate=0  xinitial=1
  Define CM Dict7 : CarMaker4SL/Define CM Dict  xname=User.IO.Out.T08.RelVyValid  xmono=off  xtype=Double4  xdvaplace=None  xnstates=0  xfirststate=0  xinitial=1
  Define CM Dict8 : CarMaker4SL/Define CM Dict  xname=User.IO.Out.T08.TypeProb  xmono=off  xtype=Double4  xdvaplace=None  xnstates=0  xfirststate=0  xinitial=1
  Define CM Dict9 : CarMaker4SL/Define CM Dict  xname=User.IO.Out.T08.Measured  xmono=off  xtype=Double4  xdvaplace=None  xnstates=0  xfirststate=0  xinitial=2

== system MIL4L3_SW6_V1_20220211/CarMaker/VehicleControl/Traffic Attribution Define1/T09 ==
  Define CM Dict 0 : CarMaker4SL/Define CM Dict  xname=User.IO.Out.T09.ExistenceProbability  xmono=off  xtype=Double4  xdvaplace=IO_Out  xnstates=0  xfirststate=0  xinitial=0.95
  Define CM Dict 1 : CarMaker4SL/Define CM Dict  xname=User.IO.Out.T09.class  xmono=off  xtype=Double4  xdvaplace=IO_Out  xnstates=0  xfirststate=0  xinitial=1
  Define CM Dict 2 : CarMaker4SL/Define CM Dict  xname=User.IO.Out.T09.ObjectInfo  xmono=off  xtype=Double4  xdvaplace=IO_Out  xnstates=0  xfirststate=0  xinitial=2
  Define CM Dict 3 : CarMaker4SL/Define CM Dict  xname=User.IO.Out.T09.ClassHighestProb  xmono=off  xtype=Double4  xdvaplace=IO_Out  xnstates=0  xfirststate=0  xinitial=2
  Define CM Dict 4 : CarMaker4SL/Define CM Dict  xname=User.IO.Out.T09.status  xmono=off  xtype=Double4  xdvaplace=IO_Out  xnstates=0  xfirststate=0  xinitial=0
  Define CM Dict 5 : CarMaker4SL/Define CM Dict  xname=User.IO.Out.T09.probility  xmono=off  xtype=Double4  xdvaplace=IO_Out  xnstates=0  xfirststate=0  xinitial=0.9
  Define CM Dict 6 : CarMaker4SL/Define CM Dict  xname=User.IO.Out.T09.power  xmono=off  xtype=Double4  xdvaplace=IO_Out  xnstates=0  xfirststate=0  xinitial=90
  Define CM Dict 7 : CarMaker4SL/Define CM Dict  xname=User.IO.Out.T09.Turn_signal  xmono=off  xtype=Double4  xdvaplace=IO_Out  xnstates=0  xfirststate=0  xinitial=0
  Define CM Dict 8 : CarMaker4SL/Define CM Dict  xname=User.IO.Out.T09.BrakeLight  xmono=off  xtype=Double4  xdvaplace=IO_Out  xnstates=0  xfirststate=0  xinitial=0
  Define CM Dict5 : CarMaker4SL/Define CM Dict  xname=User.IO.Out.T09.longdistance  xmono=off  xtype=Double4  xdvaplace=None  xnstates=0  xfirststate=0  xinitial=0
  Define CM Dict6 : CarMaker4SL/Define CM Dict  xname=User.IO.Out.T09.RelVxValid  xmono=off  xtype=Double4  xdvaplace=None  xnstates=0  xfirststate=0  xinitial=1
  Define CM Dict7 : CarMaker4SL/Define CM Dict  xname=User.IO.Out.T09.RelVyValid  xmono=off  xtype=Double4  xdvaplace=None  xnstates=0  xfirststate=0  xinitial=1
  Define CM Dict8 : CarMaker4SL/Define CM Dict  xname=User.IO.Out.T09.TypeProb  xmono=off  xtype=Double4  xdvaplace=None  xnstates=0  xfirststate=0  xinitial=1
  Define CM Dict9 : CarMaker4SL/Define CM Dict  xname=User.IO.Out.T09.Measured  xmono=off  xtype=Double4  xdvaplace=None  xnstates=0  xfirststate=0  xinitial=2

== system MIL4L3_SW6_V1_20220211/CarMaker/VehicleControl/Traffic Attribution Define1/T10 ==
  Define CM Dict 0 : CarMaker4SL/Define CM Dict  xname=User.IO.Out.T10.ExistenceProbability  xmono=off  xtype=Double4  xdvaplace=IO_Out  xnstates=0  xfirststate=0  xinitial=0.95
  Define CM Dict 1 : CarMaker4SL/Define CM Dict  xname=User.IO.Out.T10.class  xmono=off  xtype=Double4  xdvaplace=IO_Out  xnstates=0  xfirststate=0  xinitial=1
  Define CM Dict 2 : CarMaker4SL/Define CM Dict  xname=User.IO.Out.T10.ObjectInfo  xmono=off  xtype=Double4  xdvaplace=IO_Out  xnstates=0  xfirststate=0  xinitial=2
  Define CM Dict 3 : CarMaker4SL/Define CM Dict  xname=User.IO.Out.T10.ClassHighestProb  xmono=off  xtype=Double4  xdvaplace=IO_Out  xnstates=0  xfirststate=0  xinitial=2
  Define CM Dict 4 : CarMaker4SL/Define CM Dict  xname=User.IO.Out.T10.status  xmono=off  xtype=Double4  xdvaplace=IO_Out  xnstates=0  xfirststate=0  xinitial=0
  Define CM Dict 5 : CarMaker4SL/Define CM Dict  xname=User.IO.Out.T10.probility  xmono=off  xtype=Double4  xdvaplace=IO_Out  xnstates=0  xfirststate=0  xinitial=0.9
  Define CM Dict 6 : CarMaker4SL/Define CM Dict  xname=User.IO.Out.T10.power  xmono=off  xtype=Double4  xdvaplace=IO_Out  xnstates=0  xfirststate=0  xinitial=90
  Define CM Dict 7 : CarMaker4SL/Define CM Dict  xname=User.IO.Out.T10.Turn_signal  xmono=off  xtype=Double4  xdvaplace=IO_Out  xnstates=0  xfirststate=0  xinitial=0
  Define CM Dict 8 : CarMaker4SL/Define CM Dict  xname=User.IO.Out.T10.BrakeLight  xmono=off  xtype=Double4  xdvaplace=IO_Out  xnstates=0  xfirststate=0  xinitial=0
  Define CM Dict5 : CarMaker4SL/Define CM Dict  xname=User.IO.Out.T10.longdistance  xmono=off  xtype=Double4  xdvaplace=None  xnstates=0  xfirststate=0  xinitial=0
  Define CM Dict6 : CarMaker4SL/Define CM Dict  xname=User.IO.Out.T10.RelVxValid  xmono=off  xtype=Double4  xdvaplace=None  xnstates=0  xfirststate=0  xinitial=1
  Define CM Dict7 : CarMaker4SL/Define CM Dict  xname=User.IO.Out.T10.RelVyValid  xmono=off  xtype=Double4  xdvaplace=None  xnstates=0  xfirststate=0  xinitial=1
  Define CM Dict8 : CarMaker4SL/Define CM Dict  xname=User.IO.Out.T10.TypeProb  xmono=off  xtype=Double4  xdvaplace=None  xnstates=0  xfirststate=0  xinitial=1
  Define CM Dict9 : CarMaker4SL/Define CM Dict  xname=User.IO.Out.T10.Measured  xmono=off  xtype=Double4  xdvaplace=None  xnstates=0  xfirststate=0  xinitial=2

== system MIL4L3_SW6_V1_20220211/CarMaker/VehicleControl/Traffic Attribution Define1/T11 ==
  Define CM Dict 0 : CarMaker4SL/Define CM Dict  xname=User.IO.Out.T11.ExistenceProbability  xmono=off  xtype=Double4  xdvaplace=IO_Out  xnstates=0  xfirststate=0  xinitial=0.95
  Define CM Dict 1 : CarMaker4SL/Define CM Dict  xname=User.IO.Out.T11.class  xmono=off  xtype=Double4  xdvaplace=IO_Out  xnstates=0  xfirststate=0  xinitial=1
  Define CM Dict 2 : CarMaker4SL/Define CM Dict  xname=User.IO.Out.T11.ObjectInfo  xmono=off  xtype=Double4  xdvaplace=IO_Out  xnstates=0  xfirststate=0  xinitial=2
  Define CM Dict 3 : CarMaker4SL/Define CM Dict  xname=User.IO.Out.T11.ClassHighestProb  xmono=off  xtype=Double4  xdvaplace=IO_Out  xnstates=0  xfirststate=0  xinitial=2
  Define CM Dict 4 : CarMaker4SL/Define CM Dict  xname=User.IO.Out.T11.status  xmono=off  xtype=Double4  xdvaplace=IO_Out  xnstates=0  xfirststate=0  xinitial=0
  Define CM Dict 5 : CarMaker4SL/Define CM Dict  xname=User.IO.Out.T11.probility  xmono=off  xtype=Double4  xdvaplace=IO_Out  xnstates=0  xfirststate=0  xinitial=0.9
  Define CM Dict 6 : CarMaker4SL/Define CM Dict  xname=User.IO.Out.T11.power  xmono=off  xtype=Double4  xdvaplace=IO_Out  xnstates=0  xfirststate=0  xinitial=90
  Define CM Dict 7 : CarMaker4SL/Define CM Dict  xname=User.IO.Out.T11.Turn_signal  xmono=off  xtype=Double4  xdvaplace=IO_Out  xnstates=0  xfirststate=0  xinitial=0
  Define CM Dict 8 : CarMaker4SL/Define CM Dict  xname=User.IO.Out.T11.BrakeLight  xmono=off  xtype=Double4  xdvaplace=IO_Out  xnstates=0  xfirststate=0  xinitial=0
  Define CM Dict5 : CarMaker4SL/Define CM Dict  xname=User.IO.Out.T11.longdistance  xmono=off  xtype=Double4  xdvaplace=None  xnstates=0  xfirststate=0  xinitial=0
  Define CM Dict6 : CarMaker4SL/Define CM Dict  xname=User.IO.Out.T11.RelVxValid  xmono=off  xtype=Double4  xdvaplace=None  xnstates=0  xfirststate=0  xinitial=1
  Define CM Dict7 : CarMaker4SL/Define CM Dict  xname=User.IO.Out.T11.RelVyValid  xmono=off  xtype=Double4  xdvaplace=None  xnstates=0  xfirststate=0  xinitial=1
  Define CM Dict8 : CarMaker4SL/Define CM Dict  xname=User.IO.Out.T11.TypeProb  xmono=off  xtype=Double4  xdvaplace=None  xnstates=0  xfirststate=0  xinitial=1
  Define CM Dict9 : CarMaker4SL/Define CM Dict  xname=User.IO.Out.T11.Measured  xmono=off  xtype=Double4  xdvaplace=None  xnstates=0  xfirststate=0  xinitial=2

== system MIL4L3_SW6_V1_20220211/CarMaker/VehicleControl/Traffic Attribution Define1/T12 ==
  Define CM Dict 0 : CarMaker4SL/Define CM Dict  xname=User.IO.Out.T12.ExistenceProbability  xmono=off  xtype=Double4  xdvaplace=IO_Out  xnstates=0  xfirststate=0  xinitial=0.95
  Define CM Dict 1 : CarMaker4SL/Define CM Dict  xname=User.IO.Out.T12.class  xmono=off  xtype=Double4  xdvaplace=IO_Out  xnstates=0  xfirststate=0  xinitial=1
  Define CM Dict 2 : CarMaker4SL/Define CM Dict  xname=User.IO.Out.T12.ObjectInfo  xmono=off  xtype=Double4  xdvaplace=IO_Out  xnstates=0  xfirststate=0  xinitial=2
  Define CM Dict 3 : CarMaker4SL/Define CM Dict  xname=User.IO.Out.T12.ClassHighestProb  xmono=off  xtype=Double4  xdvaplace=IO_Out  xnstates=0  xfirststate=0  xinitial=2
  Define CM Dict 4 : CarMaker4SL/Define CM Dict  xname=User.IO.Out.T12.status  xmono=off  xtype=Double4  xdvaplace=IO_Out  xnstates=0  xfirststate=0  xinitial=0
  Define CM Dict 5 : CarMaker4SL/Define CM Dict  xname=User.IO.Out.T12.probility  xmono=off  xtype=Double4  xdvaplace=IO_Out  xnstates=0  xfirststate=0  xinitial=0.9
  Define CM Dict 6 : CarMaker4SL/Define CM Dict  xname=User.IO.Out.T12.power  xmono=off  xtype=Double4  xdvaplace=IO_Out  xnstates=0  xfirststate=0  xinitial=90
  Define CM Dict 7 : CarMaker4SL/Define CM Dict  xname=User.IO.Out.T12.Turn_signal  xmono=off  xtype=Double4  xdvaplace=IO_Out  xnstates=0  xfirststate=0  xinitial=0
  Define CM Dict 8 : CarMaker4SL/Define CM Dict  xname=User.IO.Out.T12.BrakeLight  xmono=off  xtype=Double4  xdvaplace=IO_Out  xnstates=0  xfirststate=0  xinitial=0
  Define CM Dict5 : CarMaker4SL/Define CM Dict  xname=User.IO.Out.T12.longdistance  xmono=off  xtype=Double4  xdvaplace=None  xnstates=0  xfirststate=0  xinitial=0
  Define CM Dict6 : CarMaker4SL/Define CM Dict  xname=User.IO.Out.T12.RelVxValid  xmono=off  xtype=Double4  xdvaplace=None  xnstates=0  xfirststate=0  xinitial=1
  Define CM Dict7 : CarMaker4SL/Define CM Dict  xname=User.IO.Out.T12.RelVyValid  xmono=off  xtype=Double4  xdvaplace=None  xnstates=0  xfirststate=0  xinitial=1
  Define CM Dict8 : CarMaker4SL/Define CM Dict  xname=User.IO.Out.T12.TypeProb  xmono=off  xtype=Double4  xdvaplace=None  xnstates=0  xfirststate=0  xinitial=1
  Define CM Dict9 : CarMaker4SL/Define CM Dict  xname=User.IO.Out.T12.Measured  xmono=off  xtype=Double4  xdvaplace=None  xnstates=0  xfirststate=0  xinitial=2

== system MIL4L3_SW6_V1_20220211/CarMaker/VehicleControl/Traffic Attribution Define1/T13 ==
  Define CM Dict 0 : CarMaker4SL/Define CM Dict  xname=User.IO.Out.T13.ExistenceProbability  xmono=off  xtype=Double4  xdvaplace=IO_Out  xnstates=0  xfirststate=0  xinitial=0.95
  Define CM Dict 1 : CarMaker4SL/Define CM Dict  xname=User.IO.Out.T13.class  xmono=off  xtype=Double4  xdvaplace=IO_Out  xnstates=0  xfirststate=0  xinitial=1
  Define CM Dict 2 : CarMaker4SL/Define CM Dict  xname=User.IO.Out.T13.ObjectInfo  xmono=off  xtype=Double4  xdvaplace=IO_Out  xnstates=0  xfirststate=0  xinitial=2
  Define CM Dict 3 : CarMaker4SL/Define CM Dict  xname=User.IO.Out.T13.ClassHighestProb  xmono=off  xtype=Double4  xdvaplace=IO_Out  xnstates=0  xfirststate=0  xinitial=2
  Define CM Dict 4 : CarMaker4SL/Define CM Dict  xname=User.IO.Out.T13.status  xmono=off  xtype=Double4  xdvaplace=IO_Out  xnstates=0  xfirststate=0  xinitial=0
  Define CM Dict 5 : CarMaker4SL/Define CM Dict  xname=User.IO.Out.T13.probility  xmono=off  xtype=Double4  xdvaplace=IO_Out  xnstates=0  xfirststate=0  xinitial=0.9
  Define CM Dict 6 : CarMaker4SL/Define CM Dict  xname=User.IO.Out.T13.power  xmono=off  xtype=Double4  xdvaplace=IO_Out  xnstates=0  xfirststate=0  xinitial=90
  Define CM Dict 7 : CarMaker4SL/Define CM Dict  xname=User.IO.Out.T13.Turn_signal  xmono=off  xtype=Double4  xdvaplace=IO_Out  xnstates=0  xfirststate=0  xinitial=0
  Define CM Dict 8 : CarMaker4SL/Define CM Dict  xname=User.IO.Out.T13.BrakeLight  xmono=off  xtype=Double4  xdvaplace=IO_Out  xnstates=0  xfirststate=0  xinitial=0
  Define CM Dict5 : CarMaker4SL/Define CM Dict  xname=User.IO.Out.T13.longdistance  xmono=off  xtype=Double4  xdvaplace=None  xnstates=0  xfirststate=0  xinitial=0
  Define CM Dict6 : CarMaker4SL/Define CM Dict  xname=User.IO.Out.T13.RelVxValid  xmono=off  xtype=Double4  xdvaplace=None  xnstates=0  xfirststate=0  xinitial=1
  Define CM Dict7 : CarMaker4SL/Define CM Dict  xname=User.IO.Out.T13.RelVyValid  xmono=off  xtype=Double4  xdvaplace=None  xnstates=0  xfirststate=0  xinitial=1
  Define CM Dict8 : CarMaker4SL/Define CM Dict  xname=User.IO.Out.T13.TypeProb  xmono=off  xtype=Double4  xdvaplace=None  xnstates=0  xfirststate=0  xinitial=1
  Define CM Dict9 : CarMaker4SL/Define CM Dict  xname=User.IO.Out.T13.Measured  xmono=off  xtype=Double4  xdvaplace=None  xnstates=0  xfirststate=0  xinitial=2

== system MIL4L3_SW6_V1_20220211/CarMaker/VehicleControl/Traffic Attribution Define1/T14 ==
  Define CM Dict 0 : CarMaker4SL/Define CM Dict  xname=User.IO.Out.T14.ExistenceProbability  xmono=off  xtype=Double4  xdvaplace=IO_Out  xnstates=0  xfirststate=0  xinitial=0.95
  Define CM Dict 1 : CarMaker4SL/Define CM Dict  xname=User.IO.Out.T14.class  xmono=off  xtype=Double4  xdvaplace=IO_Out  xnstates=0  xfirststate=0  xinitial=1
  Define CM Dict 2 : CarMaker4SL/Define CM Dict  xname=User.IO.Out.T14.ObjectInfo  xmono=off  xtype=Double4  xdvaplace=IO_Out  xnstates=0  xfirststate=0  xinitial=2
  Define CM Dict 3 : CarMaker4SL/Define CM Dict  xname=User.IO.Out.T14.ClassHighestProb  xmono=off  xtype=Double4  xdvaplace=IO_Out  xnstates=0  xfirststate=0  xinitial=2
  Define CM Dict 4 : CarMaker4SL/Define CM Dict  xname=User.IO.Out.T14.status  xmono=off  xtype=Double4  xdvaplace=IO_Out  xnstates=0  xfirststate=0  xinitial=0
  Define CM Dict 5 : CarMaker4SL/Define CM Dict  xname=User.IO.Out.T14.probility  xmono=off  xtype=Double4  xdvaplace=IO_Out  xnstates=0  xfirststate=0  xinitial=0.9
  Define CM Dict 6 : CarMaker4SL/Define CM Dict  xname=User.IO.Out.T14.power  xmono=off  xtype=Double4  xdvaplace=IO_Out  xnstates=0  xfirststate=0  xinitial=90
  Define CM Dict 7 : CarMaker4SL/Define CM Dict  xname=User.IO.Out.T14.Turn_signal  xmono=off  xtype=Double4  xdvaplace=IO_Out  xnstates=0  xfirststate=0  xinitial=0
  Define CM Dict 8 : CarMaker4SL/Define CM Dict  xname=User.IO.Out.T14.BrakeLight  xmono=off  xtype=Double4  xdvaplace=IO_Out  xnstates=0  xfirststate=0  xinitial=0
  Define CM Dict5 : CarMaker4SL/Define CM Dict  xname=User.IO.Out.T14.longdistance  xmono=off  xtype=Double4  xdvaplace=None  xnstates=0  xfirststate=0  xinitial=0
  Define CM Dict6 : CarMaker4SL/Define CM Dict  xname=User.IO.Out.T14.RelVxValid  xmono=off  xtype=Double4  xdvaplace=None  xnstates=0  xfirststate=0  xinitial=1
  Define CM Dict7 : CarMaker4SL/Define CM Dict  xname=User.IO.Out.T14.RelVyValid  xmono=off  xtype=Double4  xdvaplace=None  xnstates=0  xfirststate=0  xinitial=1
  Define CM Dict8 : CarMaker4SL/Define CM Dict  xname=User.IO.Out.T14.TypeProb  xmono=off  xtype=Double4  xdvaplace=None  xnstates=0  xfirststate=0  xinitial=1
  Define CM Dict9 : CarMaker4SL/Define CM Dict  xname=User.IO.Out.T14.Measured  xmono=off  xtype=Double4  xdvaplace=None  xnstates=0  xfirststate=0  xinitial=2

== system MIL4L3_SW6_V1_20220211/CarMaker/VehicleControl/Traffic Attribution Define1/T15 ==
  Define CM Dict 0 : CarMaker4SL/Define CM Dict  xname=User.IO.Out.T15.ExistenceProbability  xmono=off  xtype=Double4  xdvaplace=IO_Out  xnstates=0  xfirststate=0  xinitial=0.95
  Define CM Dict 1 : CarMaker4SL/Define CM Dict  xname=User.IO.Out.T15.class  xmono=off  xtype=Double4  xdvaplace=IO_Out  xnstates=0  xfirststate=0  xinitial=1
  Define CM Dict 2 : CarMaker4SL/Define CM Dict  xname=User.IO.Out.T15.ObjectInfo  xmono=off  xtype=Double4  xdvaplace=IO_Out  xnstates=0  xfirststate=0  xinitial=2
  Define CM Dict 3 : CarMaker4SL/Define CM Dict  xname=User.IO.Out.T15.ClassHighestProb  xmono=off  xtype=Double4  xdvaplace=IO_Out  xnstates=0  xfirststate=0  xinitial=2
  Define CM Dict 4 : CarMaker4SL/Define CM Dict  xname=User.IO.Out.T15.status  xmono=off  xtype=Double4  xdvaplace=IO_Out  xnstates=0  xfirststate=0  xinitial=0
  Define CM Dict 5 : CarMaker4SL/Define CM Dict  xname=User.IO.Out.T15.probility  xmono=off  xtype=Double4  xdvaplace=IO_Out  xnstates=0  xfirststate=0  xinitial=0.9
  Define CM Dict 6 : CarMaker4SL/Define CM Dict  xname=User.IO.Out.T15.power  xmono=off  xtype=Double4  xdvaplace=IO_Out  xnstates=0  xfirststate=0  xinitial=90
  Define CM Dict 7 : CarMaker4SL/Define CM Dict  xname=User.IO.Out.T15.Turn_signal  xmono=off  xtype=Double4  xdvaplace=IO_Out  xnstates=0  xfirststate=0  xinitial=0
  Define CM Dict 8 : CarMaker4SL/Define CM Dict  xname=User.IO.Out.T15.BrakeLight  xmono=off  xtype=Double4  xdvaplace=IO_Out  xnstates=0  xfirststate=0  xinitial=0
  Define CM Dict5 : CarMaker4SL/Define CM Dict  xname=User.IO.Out.T15.longdistance  xmono=off  xtype=Double4  xdvaplace=None  xnstates=0  xfirststate=0  xinitial=0
  Define CM Dict6 : CarMaker4SL/Define CM Dict  xname=User.IO.Out.T15.RelVxValid  xmono=off  xtype=Double4  xdvaplace=None  xnstates=0  xfirststate=0  xinitial=1
  Define CM Dict7 : CarMaker4SL/Define CM Dict  xname=User.IO.Out.T15.RelVyValid  xmono=off  xtype=Double4  xdvaplace=None  xnstates=0  xfirststate=0  xinitial=1
  Define CM Dict8 : CarMaker4SL/Define CM Dict  xname=User.IO.Out.T15.TypeProb  xmono=off  xtype=Double4  xdvaplace=None  xnstates=0  xfirststate=0  xinitial=1
  Define CM Dict9 : CarMaker4SL/Define CM Dict  xname=User.IO.Out.T15.Measured  xmono=off  xtype=Double4  xdvaplace=None  xnstates=0  xfirststate=0  xinitial=2

== system MIL4L3_SW6_V1_20220211/CarMaker/VehicleControl/Traffic Attribution Define1/T16 ==
  Define CM Dict 0 : CarMaker4SL/Define CM Dict  xname=User.IO.Out.T16.ExistenceProbability  xmono=off  xtype=Double4  xdvaplace=IO_Out  xnstates=0  xfirststate=0  xinitial=0.95
  Define CM Dict 1 : CarMaker4SL/Define CM Dict  xname=User.IO.Out.T16.class  xmono=off  xtype=Double4  xdvaplace=IO_Out  xnstates=0  xfirststate=0  xinitial=1
  Define CM Dict 2 : CarMaker4SL/Define CM Dict  xname=User.IO.Out.T16.ObjectInfo  xmono=off  xtype=Double4  xdvaplace=IO_Out  xnstates=0  xfirststate=0  xinitial=2
  Define CM Dict 3 : CarMaker4SL/Define CM Dict  xname=User.IO.Out.T16.ClassHighestProb  xmono=off  xtype=Double4  xdvaplace=IO_Out  xnstates=0  xfirststate=0  xinitial=2
  Define CM Dict 4 : CarMaker4SL/Define CM Dict  xname=User.IO.Out.T16.status  xmono=off  xtype=Double4  xdvaplace=IO_Out  xnstates=0  xfirststate=0  xinitial=0
  Define CM Dict 5 : CarMaker4SL/Define CM Dict  xname=User.IO.Out.T16.probility  xmono=off  xtype=Double4  xdvaplace=IO_Out  xnstates=0  xfirststate=0  xinitial=0.9
  Define CM Dict 6 : CarMaker4SL/Define CM Dict  xname=User.IO.Out.T16.power  xmono=off  xtype=Double4  xdvaplace=IO_Out  xnstates=0  xfirststate=0  xinitial=90
  Define CM Dict 7 : CarMaker4SL/Define CM Dict  xname=User.IO.Out.T16.Turn_signal  xmono=off  xtype=Double4  xdvaplace=IO_Out  xnstates=0  xfirststate=0  xinitial=0
  Define CM Dict 8 : CarMaker4SL/Define CM Dict  xname=User.IO.Out.T16.BrakeLight  xmono=off  xtype=Double4  xdvaplace=IO_Out  xnstates=0  xfirststate=0  xinitial=0
  Define CM Dict5 : CarMaker4SL/Define CM Dict  xname=User.IO.Out.T16.longdistance  xmono=off  xtype=Double4  xdvaplace=None  xnstates=0  xfirststate=0  xinitial=0
  Define CM Dict6 : CarMaker4SL/Define CM Dict  xname=User.IO.Out.T16.RelVxValid  xmono=off  xtype=Double4  xdvaplace=None  xnstates=0  xfirststate=0  xinitial=1
  Define CM Dict7 : CarMaker4SL/Define CM Dict  xname=User.IO.Out.T16.RelVyValid  xmono=off  xtype=Double4  xdvaplace=None  xnstates=0  xfirststate=0  xinitial=1
  Define CM Dict8 : CarMaker4SL/Define CM Dict  xname=User.IO.Out.T16.TypeProb  xmono=off  xtype=Double4  xdvaplace=None  xnstates=0  xfirststate=0  xinitial=1
  Define CM Dict9 : CarMaker4SL/Define CM Dict  xname=User.IO.Out.T16.Measured  xmono=off  xtype=Double4  xdvaplace=None  xnstates=0  xfirststate=0  xinitial=2
